simulink model "COSTEP"  (R2024b)
settings: Solver=FixedStepAuto  StartTime=0.0  StopTime=25  FixedStep=1/3600  RelTol=1e-3
model workspace (MAT data in the model file):
  AD : Simulink.Parameter (value not decoded)
  AG : Simulink.Parameter (value not decoded)
  AH : Simulink.Parameter (value not decoded)
  AV : Simulink.Parameter (value not decoded)
  AVP : Simulink.Parameter (value not decoded)
  BCHL : Simulink.Parameter (value not decoded)
  BCHV : Simulink.Parameter (value not decoded)
  BD : Simulink.Parameter (value not decoded)
  BDIST : Simulink.Parameter (value not decoded)
  BG : Simulink.Parameter (value not decoded)
  BH : Simulink.Parameter (value not decoded)
  BVP : Simulink.Parameter (value not decoded)
  CD : Simulink.Parameter (value not decoded)
  CDIST : Simulink.Parameter (value not decoded)
  CG : Simulink.Parameter (value not decoded)
  CH : Simulink.Parameter (value not decoded)
  CVP : Simulink.Parameter (value not decoded)
  DDIST : Simulink.Parameter (value not decoded)
  DIST_CONST : Simulink.Parameter (value not decoded)
  ISV : Simulink.Parameter (value not decoded)
  TLAST : Simulink.Parameter (value not decoded)
  TNEXT : Simulink.Parameter (value not decoded)
  XMW : Simulink.Parameter (value not decoded)
  XNS : Simulink.Parameter (value not decoded)
  XNS2 : Simulink.Parameter (value not decoded)
  XNS3 : Simulink.Parameter (value not decoded)
  XNSADD : Simulink.Parameter (value not decoded)
  XNSE : Simulink.Parameter (value not decoded)
symbols that are objects in the model workspace (value not decoded): AD, AG, AH, AV, AVP, BD, BG, BH, BVP, CD, CG, CH, CVP, XMW, XNS, XNS2, XNS3, XNSE
undefined symbols (not defined in the file or in its folder): magnitude, msgbox, SETPT, XMEAS, XMV
libraries: mylib x381, dspindex x31
(part 8 of 12)

== system COSTEP/Control Mode/Braatz/ 3/CONTROL 4 ==
  XMEAS(4) : Inport
  SETPT(4) : Inport  Port=2
  P Control Velocity form : mylib/Braatz Control/P Control Velocity form  Kc=GAIN4  Ts=SI4  X_0=XMV4_0  H=HIGH4
  XMV(4) : Outport  VectorParamsAs1DForOutWhenUnconnected=off
  wires:
  P Control Velocity form/1 -> XMV(4)/1
  XMEAS(4)/1 -> P Control Velocity form/2
  SETPT(4)/1 -> P Control Velocity form/1

== system COSTEP/Control Mode/Braatz/ 4/CONTROL 5 ==
  XMEAS(5) : Inport
  Constant4 : Constant  Value=SETPT5
  PI Control Measurement Velocity form : mylib/Braatz Control/PI Control Measurement Velocity form  Kc=GAIN5  Ti=TAUI5  Ts=SI5  X_0=XMV5_0  H=HIGH5
  XMV(5) : Outport  VectorParamsAs1DForOutWhenUnconnected=off
  wires:
  XMEAS(5)/1 -> PI Control Measurement Velocity form/2
  PI Control Measurement Velocity form/1 -> XMV(5)/1
  Constant4/1 -> PI Control Measurement Velocity form/1

== system COSTEP/Control Mode/Braatz/ 5/CONTROL 7 ==
  XMEAS(12) : Inport
  Constant4 : Constant  Value=SETPT7
  P Control Velocity form : mylib/Braatz Control/P Control Velocity form  Kc=GAIN7  Ts=SI7  X_0=XMV7_0  H=HIGH7
  XMV(7) : Outport  VectorParamsAs1DForOutWhenUnconnected=off
  wires:
  P Control Velocity form/1 -> XMV(7)/1
  Constant4/1 -> P Control Velocity form/1
  XMEAS(12)/1 -> P Control Velocity form/2

== system COSTEP/Control Mode/Braatz/ 6/CONTROL 8 ==
  XMEAS(15) : Inport
  Constant4 : Constant  Value=SETPT8
  P Control Velocity form : mylib/Braatz Control/P Control Velocity form  Kc=GAIN8  Ts=SI8  X_0=XMV8_0  H=HIGH8
  XMV(8) : Outport  VectorParamsAs1DForOutWhenUnconnected=off
  wires:
  P Control Velocity form/1 -> XMV(8)/1
  Constant4/1 -> P Control Velocity form/1
  XMEAS(15)/1 -> P Control Velocity form/2

== system COSTEP/Control Mode/Braatz/ 7/CONTROL 11 ==
  XMEAS(17) : Inport
  Constant4 : Constant  Value=SETPT11
  PI Control Measurement Velocity form : mylib/Braatz Control/PI Control Measurement Velocity form  Kc=GAIN11  Ti=TAUI11  Ts=SI11  X_0=XMV11_0  H=HIGH11
  XMV(11) : Outport  VectorParamsAs1DForOutWhenUnconnected=off
  wires:
  PI Control Measurement Velocity form/1 -> XMV(11)/1
  Constant4/1 -> PI Control Measurement Velocity form/1
  XMEAS(17)/1 -> PI Control Measurement Velocity form/2

== system COSTEP/Control Mode/Braatz/ 8/CONTROL 10 ==
  XMEAS(21) : Inport
  SETPT(10) : Inport  Port=2
  PI Control Measurement Velocity form : mylib/Braatz Control/PI Control Measurement Velocity form  Kc=GAIN10  Ti=TAUI10  Ts=SI10  X_0=XMV10_0  H=HIGH10
  XMV(10) : Outport  VectorParamsAs1DForOutWhenUnconnected=off
  wires:
  PI Control Measurement Velocity form/1 -> XMV(10)/1
  SETPT(10)/1 -> PI Control Measurement Velocity form/1
  XMEAS(21)/1 -> PI Control Measurement Velocity form/2

== system COSTEP/Control Mode/Braatz/ 8/CONTROL 18 ==
  XMEAS(9) : Inport
  Constant : Constant  Value=SETPT18
  PI Control Setpoint Velocity form : mylib/Braatz Control/PI Control Setpoint Velocity form  Kc=GAIN18  Ti=TAUI18  Ts=SI18  X_0=SETPT10  H=HIGH10  HS=HIGH18
  SETPT(10) : Outport  VectorParamsAs1DForOutWhenUnconnected=off
  wires:
  Constant/1 -> PI Control Setpoint Velocity form/1
  XMEAS(9)/1 -> PI Control Setpoint Velocity form/2
  PI Control Setpoint Velocity form/1 -> SETPT(10)/1

== system COSTEP/Control Mode/Braatz/ 9/CONTROL 16 ==
  XMEAS(18) : Inport
  SETPT(16) : Inport  Port=2
  PI Control Setpoint Velocity form : mylib/Braatz Control/PI Control Setpoint Velocity form  Kc=GAIN16  Ti=TAUI16  Ts=SI16  X_0=SETPT9  H=HIGH9  HS=HIGH16
  SETPT(9) : Outport  VectorParamsAs1DForOutWhenUnconnected=off
  wires:
  SETPT(16)/1 -> PI Control Setpoint Velocity form/1
  XMEAS(18)/1 -> PI Control Setpoint Velocity form/2
  PI Control Setpoint Velocity form/1 -> SETPT(9)/1

== system COSTEP/Control Mode/Braatz/ 9/CONTROL 20 ==
  XMEAS(38) : Inport
  Constant : Constant  Value=SETPT20
  PI Control Setpoint Velocity form : mylib/Braatz Control/PI Control Setpoint Velocity form  Kc=GAIN20  Ti=TAUI20  Ts=SI20  X_0=SETPT16  H=HIGH16  HS=HIGH20
  SETPT(16) : Outport  VectorParamsAs1DForOutWhenUnconnected=off
  wires:
  Constant/1 -> PI Control Setpoint Velocity form/1
  XMEAS(38)/1 -> PI Control Setpoint Velocity form/2
  PI Control Setpoint Velocity form/1 -> SETPT(16)/1

== system COSTEP/Control Mode/Braatz/ 9/CONTROL 9 ==
  XMEAS(19) : Inport
  SETPT(9) : Inport  Port=2
  P Control Velocity form : mylib/Braatz Control/P Control Velocity form  Kc=GAIN9  Ts=SI9  X_0=XMV9_0  H=HIGH9
  XMV(9) : Outport  VectorParamsAs1DForOutWhenUnconnected=off
  wires:
  SETPT(9)/1 -> P Control Velocity form/1
  P Control Velocity form/1 -> XMV(9)/1
  XMEAS(19)/1 -> P Control Velocity form/2

== system COSTEP/Mixing Zone/Stream 6/Subsystem/If Action Subsystem ==
  In1 : Inport
  Action Port : ActionPort  ActionPortLabel=if(u1 < 0)
  Out1 : Outport  VectorParamsAs1DForOutWhenUnconnected=off
  wires:
  In1/1 -> Out1/1

== system COSTEP/Mixing Zone/Stream 6/Subsystem/If Action Subsystem1 ==
  In1 : Inport
  Action Port : ActionPort  ActionPortLabel=else
  Out1 : Outport  VectorParamsAs1DForOutWhenUnconnected=off
  wires:
  In1/1 -> Out1/1

== system COSTEP/Process Measurements/Feed Streams/D Feed/XMWS(1) Molecular weight of Stream 1 lb//lb-mol ==
  XST(I,1) : Inport
  Product : Product
  Sum of Elements : Sum  Inputs=+
  "XMW(I) Molecular weight of components lb/lb-mol " : Constant  Value=XMW
  XMWS(1) : Outport  VectorParamsAs1DForOutWhenUnconnected=off
  wires:
  Sum of Elements/1 -> XMWS(1)/1
  Product/1 -> Sum of Elements/1
  XST(I,1)/1 -> Product/1
  "XMW(I) Molecular weight of components lb/lb-mol "/1 -> Product/2

== system COSTEP/Process Measurements/Feed Streams/E Feed/XMWS(2) Molecular weight of Stream 2 lb//lb-mol ==
  XST(I,2) : Inport
  Product : Product
  Sum of Elements : Sum  Inputs=+
  "XMW(I) Molecular weight of components lb/lb-mol " : Constant  Value=XMW
  XMWS(2) : Outport  VectorParamsAs1DForOutWhenUnconnected=off
  wires:
  Sum of Elements/1 -> XMWS(2)/1
  Product/1 -> Sum of Elements/1
  XST(I,2)/1 -> Product/1
  "XMW(I) Molecular weight of components lb/lb-mol "/1 -> Product/2

== system COSTEP/Process Measurements/Product analysis/Subsystem/Subsystem ==
  XST : Inport
  Constant : Constant  Value=100
  Multiport Selector : dspindex/Multiport Selector  rowsOrCols=Rows  idxCellArray={4,5,6,7,8}  idxErrMode=Clip Index
  XCMP(37) : Product
  XCMP(38) : Product
  XCMP(39) : Product
  XCMP(40) : Product
  XCMP(41) : Product
  "XCMP(37) " : Outport  VectorParamsAs1DForOutWhenUnconnected=off
  "XCMP(38) " : Outport  Port=2  VectorParamsAs1DForOutWhenUnconnected=off
  "XCMP(39) " : Outport  Port=3  VectorParamsAs1DForOutWhenUnconnected=off
  "XCMP(40) " : Outport  Port=4  VectorParamsAs1DForOutWhenUnconnected=off
  "XCMP(41) " : Outport  Port=5  VectorParamsAs1DForOutWhenUnconnected=off
  wires:
  Constant/1 -> XCMP(38)/2, XCMP(40)/2, XCMP(41)/2, XCMP(39)/2, XCMP(37)/2
  Multiport Selector/1 -> XCMP(37)/1
  XCMP(37)/1 -> "XCMP(37) "/1  "XCMP(37)"
  Multiport Selector/5 -> XCMP(41)/1
  XCMP(39)/1 -> "XCMP(39) "/1  "XCMP(39)"
  XST/1 -> Multiport Selector/1
  Multiport Selector/4 -> XCMP(40)/1
  Multiport Selector/2 -> XCMP(38)/1
  Multiport Selector/3 -> XCMP(39)/1
  XCMP(38)/1 -> "XCMP(38) "/1  "XCMP(38)"
  XCMP(41)/1 -> "XCMP(41) "/1  "XCMP(41)"
  XCMP(40)/1 -> "XCMP(40) "/1  "XCMP(40)"

== system COSTEP/Process Measurements/Purge gas analysis/Subsystem/Subsystem ==
  XST : Inport
  Constant : Constant  Value=100
  Multiport Selector : dspindex/Multiport Selector  rowsOrCols=Rows  idxCellArray={ 1,2,3,4,5,6,7,8}  idxErrMode=Clip Index
  XCMP(29) : Product
  XCMP(30) : Product
  XCMP(31) : Product
  XCMP(32) : Product
  XCMP(33) : Product
  XCMP(34) : Product
  XCMP(35) : Product
  XCMP(36) : Product
  "XCMP(29) " : Outport  VectorParamsAs1DForOutWhenUnconnected=off
  "XCMP(30) " : Outport  Port=2  VectorParamsAs1DForOutWhenUnconnected=off
  "XCMP(31) " : Outport  Port=3  VectorParamsAs1DForOutWhenUnconnected=off
  "XCMP(32) " : Outport  Port=4  VectorParamsAs1DForOutWhenUnconnected=off
  "XCMP(33) " : Outport  Port=5  VectorParamsAs1DForOutWhenUnconnected=off
  "XCMP(34) " : Outport  Port=6  VectorParamsAs1DForOutWhenUnconnected=off
  "XCMP(35) " : Outport  Port=7  VectorParamsAs1DForOutWhenUnconnected=off
  "XCMP(36) " : Outport  Port=8  VectorParamsAs1DForOutWhenUnconnected=off
  wires:
  XCMP(32)/1 -> "XCMP(32) "/1  "XCMP(32)"
  Multiport Selector/6 -> XCMP(34)/1
  Multiport Selector/8 -> XCMP(36)/1
  XCMP(29)/1 -> "XCMP(29) "/1  "XCMP(29)"
  Multiport Selector/5 -> XCMP(33)/1
  Multiport Selector/7 -> XCMP(35)/1
  XCMP(30)/1 -> "XCMP(30) "/1  "XCMP(30)"
  Multiport Selector/1 -> XCMP(29)/1
  Multiport Selector/3 -> XCMP(31)/1
  Constant/1 -> XCMP(32)/2, XCMP(36)/2, XCMP(35)/2, XCMP(34)/2, XCMP(33)/2, XCMP(31)/2, XCMP(30)/2, XCMP(29)/2
  XCMP(33)/1 -> "XCMP(33) "/1  "XCMP(33)"
  Multiport Selector/4 -> XCMP(32)/1
  XST/1 -> Multiport Selector/1
  Multiport Selector/2 -> XCMP(30)/1
  XCMP(31)/1 -> "XCMP(31) "/1  "XCMP(31)"
  XCMP(35)/1 -> "XCMP(35) "/1  "XCMP(35)"
  XCMP(36)/1 -> "XCMP(36) "/1  "XCMP(36)"
  XCMP(34)/1 -> "XCMP(34) "/1  "XCMP(34)"

== system COSTEP/Process Measurements/Reactor feed analysis/Subsystem/Subsystem ==
  XST : Inport
  Constant : Constant  Value=100
  Multiport Selector : dspindex/Multiport Selector  rowsOrCols=Rows  idxCellArray={ 1,2,3,4,5,6,}  idxErrMode=Clip Index
  XCMP(23) : Product
  XCMP(24) : Product
  XCMP(25) : Product
  XCMP(26) : Product
  XCMP(27) : Product
  XCMP(28) : Product
  XCMP(23)1 : Outport  VectorParamsAs1DForOutWhenUnconnected=off
  XCMP(24)1 : Outport  Port=2  VectorParamsAs1DForOutWhenUnconnected=off
  XCMP(25)1 : Outport  Port=3  VectorParamsAs1DForOutWhenUnconnected=off
  XCMP(26)1 : Outport  Port=4  VectorParamsAs1DForOutWhenUnconnected=off
  XCMP(27)1 : Outport  Port=5  VectorParamsAs1DForOutWhenUnconnected=off
  XCMP(28)1 : Outport  Port=6  VectorParamsAs1DForOutWhenUnconnected=off
  wires:
  Multiport Selector/1 -> XCMP(23)/1  "XST(1;7)"
  Multiport Selector/4 -> XCMP(26)/1  "XST(4;7)"
  Constant/1 -> XCMP(26)/2, XCMP(28)/2, XCMP(27)/2, XCMP(25)/2, XCMP(24)/2, XCMP(23)/2
  Multiport Selector/2 -> XCMP(24)/1  "XST(2;7)"
  XST/1 -> Multiport Selector/1
  Multiport Selector/6 -> XCMP(28)/1  "XST(6:7)"
  Multiport Selector/3 -> XCMP(25)/1  "XST(3;7)"
  XCMP(23)/1 -> XCMP(23)1/1  "XCMP(23)"
  Multiport Selector/5 -> XCMP(27)/1  "XST(5;7)"
  XCMP(25)/1 -> XCMP(25)1/1  "XCMP(25)"
  XCMP(26)/1 -> XCMP(26)1/1  "XCMP(26)"
  XCMP(24)/1 -> XCMP(24)1/1  "XCMP(24)"
  XCMP(27)/1 -> XCMP(27)1/1  "XCMP(27)"
  XCMP(28)/1 -> XCMP(28)1/1  "XCMP(28)"

== system COSTEP/Random number generator/Stream Measurements SMEAS Gas analysis1/Gas Analysis Delay/Subsystem ==
  In1 : Inport
  In2 : Inport  Port=2
  If : If  NumInputs=2  IfExpression=u1 == u2
  If Action Subsystem : Subsystem  TreatAsAtomicUnit=on
  If Action Subsystem1 : Subsystem  TreatAsAtomicUnit=on
  Rounding Function : Rounding  Operator=round
  Out1 : Outport  VectorParamsAs1DForOutWhenUnconnected=off
  Out2 : Outport  Port=2  VectorParamsAs1DForOutWhenUnconnected=off
  wires:
  Rounding Function/1 -> If/1, If Action Subsystem1/1(In1)
  In2/1 -> If/2
  If Action Subsystem/1(Out1) -> Out1/1
  If Action Subsystem1/1(Out1) -> Out2/1
  In1/1 -> Rounding Function/1
  If/1 -> If Action Subsystem/Action
  If/2 -> If Action Subsystem1/Action

== system COSTEP/Random number generator/Stream Measurements SMEAS Gas analysis1/If Action Subsystem3/Subsystem ==
  G : Inport
  Bus Creator2 : BusCreator  Inputs=9
  Stream 1 : Subsystem
  Stream 13 : Subsystem
  Stream 2 : Subsystem
  Stream 3 : Subsystem
  Stream 4 : Subsystem
  Stream 5 : Subsystem
  Stream 6 : Subsystem
  Stream 8 : Subsystem
  Stream 9 : Subsystem
  XMNSE2 : Outport  VectorParamsAs1DForOutWhenUnconnected=off
  G_NEW : Outport  Port=2  VectorParamsAs1DForOutWhenUnconnected=off
  wires:
  Bus Creator2/1 -> XMNSE2/1
  G/1 -> Stream 1/1(G)
  Stream 1/1(Stream 1) -> Bus Creator2/1
  Stream 1/2(G_NEW) -> Stream 2/1(G)
  Stream 2/1(Stream 2) -> Bus Creator2/2
  Stream 2/2(G_NEW) -> Stream 3/1(G)
  Stream 3/1(Stream 3) -> Bus Creator2/3
  Stream 3/2(G_NEW) -> Stream 4/1(G)
  Stream 4/1(Stream 4) -> Bus Creator2/4
  Stream 4/2(G_NEW) -> Stream 5/1(G)
  Stream 5/1(Stream 5) -> Bus Creator2/5
  Stream 5/2(G_NEW) -> Stream 6/1(G)
  Stream 6/1(Stream 6) -> Bus Creator2/6
  Stream 6/2(G_NEW) -> Stream 8/1(G)
  Stream 8/1(Stream 8) -> Bus Creator2/7
  Stream 8/2(G_NEW) -> Stream 9/1(G)
  Stream 9/1(Stream 9) -> Bus Creator2/8
  Stream 9/2(G_NEW) -> Stream 13/1(G)
  Stream 13/2(G_NEW) -> G_NEW/1
  Stream 13/1(Stream 13) -> Bus Creator2/9

== system COSTEP/Random number generator/Stream Measurements SMEAS Gas analysis1/Subsystem/If Action Subsystem ==
  In1 : Inport
  Action Port : ActionPort  ActionPortLabel=if(u1 == 0)
  Out1 : Outport  VectorParamsAs1DForOutWhenUnconnected=off
  wires:
  In1/1 -> Out1/1

== system COSTEP/Random number generator/Stream Measurements SMEAS Gas analysis1/Subsystem/If Action Subsystem1 ==
  In1 : Inport
  Action Port : ActionPort  ActionPortLabel=else
  Out1 : Outport  VectorParamsAs1DForOutWhenUnconnected=off
  wires:
  In1/1 -> Out1/1

== system COSTEP/Random number generator/Stream Measurements SMEAS Product analysis1/Gas Analysis Delay/Subsystem ==
  In1 : Inport
  In2 : Inport  Port=2
  If : If  NumInputs=2  IfExpression=u1 == u2
  If Action Subsystem : Subsystem  TreatAsAtomicUnit=on
  If Action Subsystem1 : Subsystem  TreatAsAtomicUnit=on
  Rounding Function : Rounding  Operator=round
  Out1 : Outport  VectorParamsAs1DForOutWhenUnconnected=off
  Out2 : Outport  Port=2  VectorParamsAs1DForOutWhenUnconnected=off
  wires:
  Rounding Function/1 -> If/1, If Action Subsystem1/1(In1)
  In2/1 -> If/2
  If Action Subsystem/1(Out1) -> Out1/1
  If Action Subsystem1/1(Out1) -> Out2/1
  In1/1 -> Rounding Function/1
  If/1 -> If Action Subsystem/Action
  If/2 -> If Action Subsystem1/Action

== system COSTEP/Random number generator/Stream Measurements SMEAS Product analysis1/If Action Subsystem3/Subsystem ==
  G : Inport
  Bus Creator : BusCreator  Inputs=2
  Subsystem1 : Subsystem
  Subsystem2 : Subsystem
  XMNSE3 : Outport  VectorParamsAs1DForOutWhenUnconnected=off
  G_NEW : Outport  Port=2  VectorParamsAs1DForOutWhenUnconnected=off
  wires:
  G/1 -> Subsystem1/1(G)
  Subsystem1/1(Stream 11) -> Bus Creator/1
  Bus Creator/1 -> XMNSE3/1
  Subsystem1/2(G_NEW) -> Subsystem2/1(G)
  Subsystem2/1(Stream 13) -> Bus Creator/2
  Subsystem2/2(G_NEW) -> G_NEW/1

== system COSTEP/Random number generator/Stream Measurements SMEAS Product analysis1/Subsystem/If Action Subsystem ==
  In1 : Inport
  Action Port : ActionPort  ActionPortLabel=if(u1 == 0)
  Out1 : Outport  VectorParamsAs1DForOutWhenUnconnected=off
  wires:
  In1/1 -> Out1/1

== system COSTEP/Random number generator/Stream Measurements SMEAS Product analysis1/Subsystem/If Action Subsystem1 ==
  In1 : Inport
  Action Port : ActionPort  ActionPortLabel=else
  Out1 : Outport  VectorParamsAs1DForOutWhenUnconnected=off
  wires:
  In1/1 -> Out1/1

== system COSTEP/Reactor/Reaction Rates/Component reaction rate lb-mol//h/Subsystem ==
  RR : Inport
  " " : Sum  Inputs=---
  Bus Selector : BusSelector  OutputSignals=RR(1),RR(2),RR(3)
  CRXR(1) : Outport  VectorParamsAs1DForOutWhenUnconnected=off
  wires:
  " "/1 -> CRXR(1)/1  "CRXR(1)"
  Bus Selector/2 -> " "/2  "<RR(2)>"
  Bus Selector/3 -> " "/3  "<RR(3)>"
  RR/1 -> Bus Selector/1
  Bus Selector/1 -> " "/1  "<RR(1)>"

== system COSTEP/Reactor/Reaction Rates/Component reaction rate lb-mol//h/Subsystem1 ==
  RR : Inport
  " " : Sum  Inputs=--
  Bus Selector : BusSelector  OutputSignals=RR(1),RR(2)
  CRXR(3) : Outport  VectorParamsAs1DForOutWhenUnconnected=off
  wires:
  " "/1 -> CRXR(3)/1  "CRXR(3)"
  RR/1 -> Bus Selector/1
  Bus Selector/1 -> " "/1  "<RR(1)>"
  Bus Selector/2 -> " "/2  "<RR(2)>"

== system COSTEP/Reactor/Reaction Rates/Component reaction rate lb-mol//h/Subsystem2 ==
  RR : Inport
  " " : Sum  Inputs=--
  Bus Selector : BusSelector  OutputSignals=RR(1),RR(4)
  Gain : Gain  Gain=1.5
  CRXR(4) : Outport  VectorParamsAs1DForOutWhenUnconnected=off
  wires:
  Gain/1 -> " "/2
  Bus Selector/1 -> " "/1  "<RR(1)>"
  " "/1 -> CRXR(4)/1  "CRXR(4)"
  RR/1 -> Bus Selector/1
  Bus Selector/2 -> Gain/1  "<RR(4)>"

== system COSTEP/Reactor/Reaction Rates/Component reaction rate lb-mol//h/Subsystem3 ==
  RR : Inport
  " " : Sum  Inputs=--
  Bus Selector : BusSelector  OutputSignals=RR(2),RR(3)
  CRXR(5) : Outport  VectorParamsAs1DForOutWhenUnconnected=off
  wires:
  " "/1 -> CRXR(5)/1  "CRXR(5)"
  RR/1 -> Bus Selector/1
  Bus Selector/1 -> " "/1  "<RR(2)>"
  Bus Selector/2 -> " "/2  "<RR(3)>"

== system COSTEP/Reactor/Reaction Rates/Component reaction rate lb-mol//h/Subsystem4 ==
  RR : Inport
  " " : Sum
  Bus Selector : BusSelector  OutputSignals=RR(3),RR(4)
  CRXR(6) : Outport  VectorParamsAs1DForOutWhenUnconnected=off
  wires:
  " "/1 -> CRXR(6)/1  "CRXR(6)"
  RR/1 -> Bus Selector/1
  Bus Selector/2 -> " "/2  "<RR(4)>"
  Bus Selector/1 -> " "/1  "<RR(3)>"

== system COSTEP/Reactor/Reaction Rates/Component reaction rate lb-mol//h/Subsystem5 ==
  RR : Inport
  Bus Selector : BusSelector  OutputSignals=RR(1)
  Gain : Gain
  CRXR(7) : Outport  VectorParamsAs1DForOutWhenUnconnected=off
  wires:
  Bus Selector/1 -> Gain/1  "<RR(1)>"
  RR/1 -> Bus Selector/1
  Gain/1 -> CRXR(7)/1  "CRXR(7)"

== system COSTEP/Reactor/Reaction Rates/Component reaction rate lb-mol//h/Subsystem6 ==
  RR : Inport
  " " : Gain
  Bus Selector : BusSelector  OutputSignals=RR(2)
  CRXR(8) : Outport  VectorParamsAs1DForOutWhenUnconnected=off
  wires:
  " "/1 -> CRXR(8)/1  "CRXR(8)"
  RR/1 -> Bus Selector/1
  Bus Selector/1 -> " "/1  "<RR(2)>"

== system COSTEP/Reactor/Reaction Rates/Reaction rates lb-mol//h/ Reaction rate of reaction 4 lb-mol//ft3·h     ==
  PPR : Inport
  TKR : Inport  Port=2
  Activation energy cal/mol : Constant  Value=60000
  Bus Selector : BusSelector  OutputSignals=PPR(1),PPR(4)
  Divide : Product  Inputs=*//
  Divide1 : Product  Inputs=3
  Gain : Gain  Gain=0.767488334
  Math Function2 : Math  SignedPower=on
  Preexponential factor lb-mol/ft3·h·mmHg : Constant  Value=53.4060443
  Subtract : Sum  Inputs=+-
  Universal gas constant cal/mol·K : Constant  Value=1.987
  RR(4) : Outport  VectorParamsAs1DForOutWhenUnconnected=off
  wires:
  Divide/1 -> Subtract/2
  Universal gas constant cal/mol·K/1 -> Divide/2
  Preexponential factor lb-mol/ft3·h·mmHg/1 -> Subtract/1
  Activation energy cal/mol/1 -> Divide/1
  TKR/1 -> Divide/3
  Subtract/1 -> Math Function2/1
  Divide1/1 -> RR(4)/1
  Bus Selector/2 -> Divide1/3  "<PPR(4)>"
  Gain/1 -> Divide1/1
  Math Function2/1 -> Gain/1
  PPR/1 -> Bus Selector/1
  Bus Selector/1 -> Divide1/2  "<PPR(1)>"

== system COSTEP/Reactor/Reaction Rates/Reaction rates lb-mol//h/Reaction rate of reaction 1 lb-mol//ft3·h ==
  PPR : Inport
  TKR : Inport  Port=2
  " " : Constant  Value=0
  Abs : Abs  SaturateOnIntegerOverflow=off
  Bus Selector : BusSelector  OutputSignals=PPR(1),PPR(3)
  If : If  NumInputs=2  IfExpression=u1>0 & u2>0
  If Action Subsystem : Subsystem  TreatAsAtomicUnit=on
  If Action Subsystem2 : Subsystem  TreatAsAtomicUnit=on
  Merge1 : Merge
  "RR(1) Reaction rate of 1st reaction lb-mol/ft3·h " : Subsystem
  RR(1) : Outport  VectorParamsAs1DForOutWhenUnconnected=off
  wires:
  "RR(1) Reaction rate of 1st reaction lb-mol/ft3·h "/1(RR(1)) -> If Action Subsystem/1(In1)
  If/1 -> If Action Subsystem/Action
  " "/1 -> If Action Subsystem2/1(In1)
  If/2 -> If Action Subsystem2/Action
  Merge1/1 -> Abs/1
  If Action Subsystem/1(Out1) -> Merge1/1
  If Action Subsystem2/1(Out1) -> Merge1/2
  TKR/1 -> "RR(1) Reaction rate of 1st reaction lb-mol/ft3·h "/2(TKR)
  Abs/1 -> RR(1)/1
  PPR/1 -> "RR(1) Reaction rate of 1st reaction lb-mol/ft3·h "/1(PPR), Bus Selector/1
  Bus Selector/1 -> If/1  "<PPR(1)>"
  Bus Selector/2 -> If/2  "<PPR(3)>"

== system COSTEP/Reactor/Reaction Rates/Reaction rates lb-mol//h/Reaction rate of reaction 2 lb-mol//ft3·h ==
  PPR : Inport
  TKR : Inport  Port=2
  " " : Constant  Value=0
  Abs : Abs  SaturateOnIntegerOverflow=off
  Bus Selector : BusSelector  OutputSignals=PPR(1),PPR(3)
  If : If  NumInputs=2  IfExpression=u1>0 & u2>0
  If Action Subsystem : Subsystem  TreatAsAtomicUnit=on
  If Action Subsystem2 : Subsystem  TreatAsAtomicUnit=on
  Merge1 : Merge
  "RR(2) Reaction rate of 2nd reaction lb-mol/ft3·h " : Subsystem
  RR(2) : Outport  VectorParamsAs1DForOutWhenUnconnected=off
  wires:
  If/1 -> If Action Subsystem/Action
  If/2 -> If Action Subsystem2/Action
  "RR(2) Reaction rate of 2nd reaction lb-mol/ft3·h "/1(RR(2)) -> If Action Subsystem/1(In1)
  " "/1 -> If Action Subsystem2/1(In1)
  If Action Subsystem2/1(Out1) -> Merge1/2
  TKR/1 -> "RR(2) Reaction rate of 2nd reaction lb-mol/ft3·h "/2(TKR)
  If Action Subsystem/1(Out1) -> Merge1/1
  Merge1/1 -> Abs/1
  Abs/1 -> RR(2)/1
  PPR/1 -> "RR(2) Reaction rate of 2nd reaction lb-mol/ft3·h "/1(PPR), Bus Selector/1
  Bus Selector/1 -> If/1  "<PPR(1)>"
  Bus Selector/2 -> If/2  "<PPR(3)>"

== system COSTEP/Reactor/Reaction Rates/Reaction rates lb-mol//h/Reaction rate of reaction 3 lb-mol//ft3·h   ==
  PPR : Inport
  TKR : Inport  Port=2
  Activation energy cal/mol : Constant  Value=60000
  Bus Selector : BusSelector  OutputSignals=PPR(1),PPR(5)
  Divide : Product  Inputs=*//
  Divide1 : Product  Inputs=3
  Math Function2 : Math  SignedPower=on
  Preexponential factor lb-mol/ft3·h·mmHg : Constant  Value=53.4060443
  Subtract : Sum  Inputs=+-
  Universal gas constant cal/mol·K : Constant  Value=1.987
  RR(3) : Outport  VectorParamsAs1DForOutWhenUnconnected=off
  wires:
  Divide/1 -> Subtract/2
  Universal gas constant cal/mol·K/1 -> Divide/2
  Preexponential factor lb-mol/ft3·h·mmHg/1 -> Subtract/1
  Activation energy cal/mol/1 -> Divide/1
  TKR/1 -> Divide/3
  Subtract/1 -> Math Function2/1
  Bus Selector/2 -> Divide1/3  "<PPR(5)>"
  Divide1/1 -> RR(3)/1
  Math Function2/1 -> Divide1/1
  PPR/1 -> Bus Selector/1
  Bus Selector/1 -> Divide1/2  "<PPR(1)>"

== system COSTEP/Reactor/Reactor Heat exchanger/Position of Valve 12 %/Control valve ==
  XMV(12) : Inport
  Saturation : Saturate  UpperLimit=100  LowerLimit=0
  VCV(12) : Outport  PortDimensions=1  VectorParamsAs1DForOutWhenUnconnected=off
  wires:
  Saturation/1 -> VCV(12)/1
  XMV(12)/1 -> Saturation/1

== system COSTEP/Reactor/Reactor Heat exchanger/Reactor Heat exchanger/AGSP Agitation speed ==
  VPOS(12) : Inport
  " " : Product  Inputs=*/
  Add : Sum
  Constant1 : Constant  Value=150
  Constant2 : Constant  Value=100
  AGSP : Outport  VectorParamsAs1DForOutWhenUnconnected=off
  wires:
  Constant2/1 -> " "/2
  " "/1 -> AGSP/1
  VPOS(12)/1 -> Add/1
  Constant1/1 -> Add/2
  Add/1 -> " "/1

== system COSTEP/Reactor/Reactor Heat exchanger/Reactor Heat exchanger/Cooling water outlet temperature ==
  FWR : Inport
  QUR : Inport  Port=2  PortDimensions=1
  Constant : Constant  Value=37
  Constant1 : Constant  Value=1e6
  Constant2 : Constant  Value=1.8
  Constant6 : Constant  Value=500.53
  Divide : Product  Inputs=*/
  Divide1 : Product
  Divide2 : Product  Inputs=*/
  HWR : Constant  Value=7060
  Initial state variable : mylib/Initial state variable
  Integration : mylib/Integration  SystemSampleTime=-1  VariantActivationTime=update diagram  AllowFlexibleInterface=on  Latency=0  AutoFrameSizeCalculation=off
  Product : Product  Inputs=3
  Subtract : Sum  Inputs=+-
  "TCWR Inlet temperature of cooling water °C " : Subsystem
  TCWR-TWR : Sum  Inputs=+-
  "YY(37) " : Outport  VectorParamsAs1DForOutWhenUnconnected=off
  tag scope: TCWR=global, TWR=global
  wires:
  Divide2/1 -> Integration/1
  Initial state variable/1 -> Integration/2
  "TCWR Inlet temperature of cooling water °C "/1(TCWR) -> [TCWR], TCWR-TWR/1
  Integration/1 -> TCWR-TWR/2, "YY(37) "/1, [TWR]
  FWR/1 -> Product/1
  Constant6/1 -> Product/2
  TCWR-TWR/1 -> Product/3
  QUR/1 -> Divide1/1
  Constant1/1 -> Divide1/2
  Divide1/1 -> Divide/1
  Constant2/1 -> Divide/2
  Product/1 -> Subtract/1
  Divide/1 -> Subtract/2
  Subtract/1 -> Divide2/1
  HWR/1 -> Divide2/2
  Constant/1 -> Initial state variable/1

== system COSTEP/Reactor/Reactor Heat exchanger/Reactor Heat exchanger/FWR Flow of cooling water to reactor gallons per minute ==
  VPOS(10) : Inport
  VRNG(10) : Inport  Port=2
  " " : Product  Inputs=**/
  Constant2 : Constant  Value=100
  FWR : Outport  VectorParamsAs1DForOutWhenUnconnected=off
  wires:
  Constant2/1 -> " "/3
  " "/1 -> FWR/1
  VPOS(10)/1 -> " "/1
  VRNG(10)/1 -> " "/2

== system COSTEP/Reactor/Reactor Heat exchanger/Reactor Heat exchanger/Subsystem ==
  VLR : Inport
  Constant : Constant  Value=7.8
  Constant1 : Constant
  Constant2 : Constant  Value=0
  Constant3 : Constant  Value=0.025
  Constant4 : Constant  Value=0.25
  Divide : Product  Inputs=*/
  Divide1 : Product  Inputs=**
  If : If  IfExpression=u1 > 50  ElseIfExpressions=u1 < 10
  If Action Subsystem : Subsystem  TreatAsAtomicUnit=on
  If Action Subsystem1 : Subsystem  TreatAsAtomicUnit=on
  If Action Subsystem2 : Subsystem  TreatAsAtomicUnit=on
  Subtract : Sum  Inputs=+-
  UARLEV : Merge  Inputs=3
  "UARLEV " : Outport  VectorParamsAs1DForOutWhenUnconnected=off
  wires:
  If/2 -> If Action Subsystem1/Action
  If/1 -> If Action Subsystem/Action
  UARLEV/1 -> "UARLEV "/1
  If Action Subsystem1/1(Out1) -> UARLEV/2
  If Action Subsystem/1(Out1) -> UARLEV/1
  If/3 -> If Action Subsystem2/Action
  If Action Subsystem2/1(Out1) -> UARLEV/3
  VLR/1 -> Divide/1
  Constant/1 -> Divide/2
  Divide/1 -> Divide1/2, If/1
  Constant1/1 -> If Action Subsystem/1(In1)
  Constant2/1 -> If Action Subsystem1/1(In1)
  Constant3/1 -> Divide1/1
  Divide1/1 -> Subtract/1
  Constant4/1 -> Subtract/2
  Subtract/1 -> If Action Subsystem2/1(In1)

== system COSTEP/Reactor/Reactor Heat exchanger/Reactor Heat exchanger/Subsystem2 ==
  UARLEV : Inport
  AGSP : Inport  Port=2
  Add : Sum  Inputs=++-
  Constant : Constant  Value=-0.5
  Constant1 : Constant  Value=2.75
  Constant2 : Constant  Value=2.5
  Constant3 : Constant  Value=855490E-6
  Math Function : Math  Operator=magnitude^2  SignedPower=on
  Product : Product
  Product1 : Product
  UAR : Product  Inputs=3
  "UAR " : Outport
  wires:
  Constant/1 -> Product/1
  Constant3/1 -> UAR/3
  AGSP/1 -> Product1/2, Math Function/1
  Add/1 -> UAR/2
  Product1/1 -> Add/2
  Math Function/1 -> Product/2
  Constant1/1 -> Product1/1
  Constant2/1 -> Add/3
  Product/1 -> Add/1
  UAR/1 -> "UAR "/1
  UARLEV/1 -> UAR/1

== system COSTEP/Reactor/Reactor Heat exchanger/Reactor Heat exchanger/Subsystem3 ==
  UAR : Inport
  TWR : Inport  Port=2
  TCR : Inport  Port=3
  Bus Selector : BusSelector  OutputSignals=signal2.TESUB8(10)
  Constant4 : Constant
  Constant5 : Constant  Value=0.35
  Product2 : Product
  QUR : Product  Inputs=3
  Subtract : Sum  Inputs=+-
  Subtract1 : Sum  Inputs=+-
  "QUR " : Outport
  wires:
  Product2/1 -> Subtract1/2
  UAR/1 -> QUR/1
  Subtract/1 -> QUR/2
  [TESUB8] -> Bus Selector/1
  Constant4/1 -> Subtract1/1
  Subtract1/1 -> QUR/3
  Constant5/1 -> Product2/1
  TWR/1 -> Subtract/1
  Bus Selector/1 -> Product2/2  "<TESUB8(10)>"
  TCR/1 -> Subtract/2
  QUR/1 -> "QUR "/1

== system COSTEP/Reactor/Stream 8/Subsystem/If Action Subsystem ==
  In1 : Inport
  Action Port : ActionPort  ActionPortLabel=if(u1 < 0)
  Out1 : Outport  VectorParamsAs1DForOutWhenUnconnected=off
  wires:
  In1/1 -> Out1/1

== system COSTEP/Reactor/Stream 8/Subsystem/If Action Subsystem1 ==
  In1 : Inport
  Action Port : ActionPort  ActionPortLabel=else
  Out1 : Outport  VectorParamsAs1DForOutWhenUnconnected=off
  wires:
  In1/1 -> Out1/1

== system COSTEP/Reactor/Volume of Reactor/DLR Molar Density of Liquids in Reactor lb-mol//ft³    /DLR Molar Density of Liquids in Reactor lb-mol//ft³  ==
  X : Inport
  T : Inport  Port=2
  "  " : Constant
  "    " : Product  Inputs=*/
  AD(I) : Constant  Value=AD
  Add2 : Sum
  BD(I) : Constant  Value=BD
  CD(I) : Constant  Value=CD
  Liquid Density of Components lb/ft³ : Sum
  Molecular weight of components lb/lb-mol : Constant  Value=XMW
  Product : Product
  Product1 : Product
  Product2 : Product
  Sum of Elements : Sum  Inputs=+
  V Molar Volume of Components ft³/lb-mol : Product  Inputs=*/
  "R " : Outport  VectorParamsAs1DForOutWhenUnconnected=off
  wires:
  Liquid Density of Components lb/ft³/1 -> V Molar Volume of Components ft³/lb-mol/2
  Product1/1 -> Liquid Density of Components lb/ft³/2
  T/1 -> Product1/2, Product/2
  "  "/1 -> "    "/1
  AD(I)/1 -> Liquid Density of Components lb/ft³/1
  Add2/1 -> Product1/1
  V Molar Volume of Components ft³/lb-mol/1 -> Sum of Elements/1
  CD(I)/1 -> Product/1
  Product2/1 -> V Molar Volume of Components ft³/lb-mol/1
  BD(I)/1 -> Add2/1
  Product/1 -> Add2/2
  "    "/1 -> "R "/1
  X/1 -> Product2/1
  Sum of Elements/1 -> "    "/2
  Molecular weight of components lb/lb-mol/1 -> Product2/2

== system COSTEP/Separator/Stream 10/Subsystem/If Action Subsystem ==
  In1 : Inport
  Action Port : ActionPort  ActionPortLabel=if(u1 < 0)
  Out1 : Outport  VectorParamsAs1DForOutWhenUnconnected=off
  wires:
  In1/1 -> Out1/1

== system COSTEP/Separator/Stream 10/Subsystem/If Action Subsystem1 ==
  In1 : Inport
  Action Port : ActionPort  ActionPortLabel=else
  Out1 : Outport  VectorParamsAs1DForOutWhenUnconnected=off
  wires:
  In1/1 -> Out1/1

== system COSTEP/Separator/Stream 11/PTSL Pressure of Liquid From Separator mmHg/VPR Vapour Pressure mmHg ==
  TCR : Inport
  AVP(I) Antoine Coefficient A ln(mmHg) : Constant  Value=AVP
  Add : Sum
  Add1 : Sum
  BVP(I) Antoine Coefficient B ln(mmHg)·°C : Constant  Value=BVP
  CVP(I) Antoine Coefficient C °C : Constant  Value=CVP
  Divide : Product  Inputs=*/
  Math Function : Math  SignedPower=on
  VPR : Outport  VectorParamsAs1DForOutWhenUnconnected=off
  wires:
  BVP(I) Antoine Coefficient B ln(mmHg)·°C/1 -> Divide/1
  CVP(I) Antoine Coefficient C °C/1 -> Add/1
  AVP(I) Antoine Coefficient A ln(mmHg)/1 -> Add1/1
  Add/1 -> Divide/2
  Divide/1 -> Add1/2
  Add1/1 -> Math Function/1
  Math Function/1 -> VPR/1
  TCR/1 -> Add/2

== system COSTEP/Separator/Stream 9/Subsystem/If Action Subsystem2 ==
  In1 : Inport
  Action Port : ActionPort  ActionPortLabel=if(u1 < 1E-3)
  Out1 : Outport  VectorParamsAs1DForOutWhenUnconnected=off
  wires:
  In1/1 -> Out1/1

== system COSTEP/Separator/Stream 9/Subsystem/If Action Subsystem3 ==
  In1 : Inport
  Action Port : ActionPort  ActionPortLabel=else
  Out1 : Outport  PortDimensions=1  VectorParamsAs1DForOutWhenUnconnected=off
  wires:
  In1/1 -> Out1/1

== system COSTEP/Separator/Stream 9/Subsystem/Pressure drop ==
  Constant : Constant  Value=0.0
  DLP : Sum  Inputs=+-
  DLP Pressure drop between separator and reactor : Merge
  If : If  IfExpression=u1 < 0
  If Action Subsystem : Subsystem  TreatAsAtomicUnit=on
  If Action Subsystem1 : Subsystem  TreatAsAtomicUnit=on
  "DLP " : Outport  VectorParamsAs1DForOutWhenUnconnected=off
  wires:
  DLP Pressure drop between separator and reactor/1 -> "DLP "/1
  [PTV] -> DLP/1
  Constant/1 -> If Action Subsystem/1(In1)
  DLP/1 -> If Action Subsystem1/1(In1), If/1
  If/2 -> If Action Subsystem1/Action
  If/1 -> If Action Subsystem/Action
  [PTS] -> DLP/2
  If Action Subsystem1/1(Out1) -> DLP Pressure drop between separator and reactor/2
  If Action Subsystem/1(Out1) -> DLP Pressure drop between separator and reactor/1

== system COSTEP/Separator/Volume of Separator/DLS Molar Density of Liquids in Reactor lb-mol//ft³    /DLS Molar Density of Liquids in Separator lb-mol//ft³  ==
  X : Inport
  T : Inport  Port=2
  "  " : Constant
  "    " : Product  Inputs=*/
  AD(I) : Constant  Value=AD
  Add2 : Sum
  BD(I) : Constant  Value=BD
  CD(I) : Constant  Value=CD
  Liquid Density of Components lb/ft³ : Sum
  Product : Product
  Product1 : Product
  Product2 : Product
  Sum of Elements : Sum  Inputs=+
  V Molar Volume of Components ft³/lb-mol : Product  Inputs=*/
  XMW : Constant  Value=XMW
  "R " : Outport  VectorParamsAs1DForOutWhenUnconnected=off
  wires:
  Liquid Density of Components lb/ft³/1 -> V Molar Volume of Components ft³/lb-mol/2
  Product1/1 -> Liquid Density of Components lb/ft³/2
  T/1 -> Product1/2, Product/2
  "  "/1 -> "    "/1
  AD(I)/1 -> Liquid Density of Components lb/ft³/1
  Add2/1 -> Product1/1
  V Molar Volume of Components ft³/lb-mol/1 -> Sum of Elements/1
  CD(I)/1 -> Product/1
  Product2/1 -> V Molar Volume of Components ft³/lb-mol/1
  BD(I)/1 -> Add2/1
  Product/1 -> Add2/2
  "    "/1 -> "R "/1
  X/1 -> Product2/1
  Sum of Elements/1 -> "    "/2
  XMW/1 -> Product2/2

== system COSTEP/Stream Measurements/Subsystem6/A and C feed stream/Composition measurement mol% ==
  XST : Inport
  XMNSE : Inport  Port=2
  Bus Creator : BusCreator  Inputs=3
  Subsystem : Subsystem
  SMEASX(4) : Outport
  wires:
  Subsystem/3(SMEASXC(4)) -> Bus Creator/3  "SMEASXC(4)"
  XST/1 -> Subsystem/1(XST)
  Subsystem/2(SMEASXB(4)) -> Bus Creator/2  "SMEASXB(4)"
  Subsystem/1(SMEASXA(4)) -> Bus Creator/1  "SMEASXA(4)"
  Bus Creator/1 -> SMEASX(4)/1  "SMEASX(4)"
  XMNSE/1 -> Subsystem/2(XMNSE)

== system COSTEP/Stream Measurements/Subsystem6/A and C feed stream/Flow measurement in kg//h ==
  XMEAS in kscmh : Inport
  XST : Inport  Port=2
  " " : Constant  Value=35.3145
  "  " : Constant  Value=0.359
  Convert from lb/h to kg/h : Constant  Value=0.454
  Product : Product  Inputs=3
  XMWS Molecular weight of Stream lb/lb-mol : Subsystem
  lb-mol/h : Product  Inputs=**/
  "SMEASF(4) " : Outport  VectorParamsAs1DForOutWhenUnconnected=off
  wires:
  " "/1 -> lb-mol/h/2
  "  "/1 -> lb-mol/h/3
  XMEAS in kscmh/1 -> lb-mol/h/1
  Convert from lb/h to kg/h/1 -> Product/3
  XST/1 -> XMWS Molecular weight of Stream lb/lb-mol/1(XST)
  lb-mol/h/1 -> Product/2
  XMWS Molecular weight of Stream lb/lb-mol/1(XMWS) -> Product/1
  Product/1 -> "SMEASF(4) "/1  "SMEASF(4)"

== system COSTEP/Stream Measurements/Subsystem6/A and C feed stream/Pressure measurement in kPa ==
  "P in mm Hg " : Inport
  XMNSE : Inport  Port=2
  " kPa" : Constant  Value=101.325
  " mm Hg   " : Constant  Value=760
  Add : Sum
  Pressure conversion kPa : Product  Inputs=*/*
  SMEASP(4) : Outport  VectorParamsAs1DForOutWhenUnconnected=off
  wires:
  "P in mm Hg "/1 -> Pressure conversion kPa/1
  " kPa"/1 -> Pressure conversion kPa/3
  " mm Hg   "/1 -> Pressure conversion kPa/2
  Pressure conversion kPa/1 -> Add/1
  Add/1 -> SMEASP(4)/1  "SMEASP(4)"
  XMNSE/1 -> Add/2

== system COSTEP/Stream Measurements/Subsystem6/A and C feed stream/Temperature measurement in C ==
  T in celsius : Inport
  XMNSE : Inport  Port=2
  Add : Sum
  SMEAST(4) : Outport
  wires:
  T in celsius/1 -> Add/1
  Add/1 -> SMEAST(4)/1  "SMEAST"
  XMNSE/1 -> Add/2

== system COSTEP/Stream Measurements/Subsystem6/A feed stream/Composition measurement mol% ==
  XST : Inport
  XMNSE : Inport  Port=2
  Bus Creator : BusCreator  Inputs=2
  Subsystem : Subsystem
  SMEASX(1) : Outport
  wires:
  XST/1 -> Subsystem/1(XST)
  Subsystem/2(SMEASXB(1)) -> Bus Creator/2  "SMEASXB(1)"
  Subsystem/1(SMEASXA(1)) -> Bus Creator/1  "SMEASXA(1)"
  Bus Creator/1 -> SMEASX(1)/1  "SMEASX(1)"
  XMNSE/1 -> Subsystem/2(XMNSE)

== system COSTEP/Stream Measurements/Subsystem6/A feed stream/Flow measurement in kg//h ==
  XMEAS in kscmh : Inport
  XST : Inport  Port=2
  " " : Constant  Value=35.3145
  "  " : Constant  Value=0.359
  Convert from lb/h to kg/h : Constant  Value=0.454
  XMWS Molecular weight of Stream lb/lb-mol : Subsystem
  kg/h : Product  Inputs=3
  lb-mol/h : Product  Inputs=**/
  "SMEASF(1) " : Outport  VectorParamsAs1DForOutWhenUnconnected=off
  wires:
  " "/1 -> lb-mol/h/2
  "  "/1 -> lb-mol/h/3
  XMEAS in kscmh/1 -> lb-mol/h/1
  Convert from lb/h to kg/h/1 -> kg/h/3
  XST/1 -> XMWS Molecular weight of Stream lb/lb-mol/1(XST)
  lb-mol/h/1 -> kg/h/2
  XMWS Molecular weight of Stream lb/lb-mol/1(XMWS) -> kg/h/1
  kg/h/1 -> "SMEASF(1) "/1

== system COSTEP/Stream Measurements/Subsystem6/A feed stream/Pressure measurement in kPa ==
  "P in mm Hg " : Inport
  XMNSE : Inport  Port=2
  " kPa" : Constant  Value=101.325
  " mm Hg   " : Constant  Value=760
  Add : Sum
  Pressure conversion kPa : Product  Inputs=*/*
  SMEASP(1) : Outport  VectorParamsAs1DForOutWhenUnconnected=off
  wires:
  "P in mm Hg "/1 -> Pressure conversion kPa/1
  " kPa"/1 -> Pressure conversion kPa/3
  " mm Hg   "/1 -> Pressure conversion kPa/2
  Pressure conversion kPa/1 -> Add/1
  Add/1 -> SMEASP(1)/1  "SMEASP"
  XMNSE/1 -> Add/2

== system COSTEP/Stream Measurements/Subsystem6/A feed stream/Temperature measurement in C ==
  T in celsius : Inport
  XMNSE : Inport  Port=2
  Add : Sum
  SMEAST(1) : Outport
  wires:
  T in celsius/1 -> Add/1
  Add/1 -> SMEAST(1)/1  "SMEAST"
  XMNSE/1 -> Add/2

== system COSTEP/Stream Measurements/Subsystem6/CCIn/Flow measurement in kg//h ==
  XMNSE : Inport
  F in gpm : Inport  Port=2
  Add : Sum
  Product : Product
  Product1 : Product
  gpm to lb/h : Constant  Value=500.72
  kg/kmol : Constant  Value=18.02
  kmol : Constant  Value=0.45359237
  kmol/h : Product
  lb/h to lb-mol/h : Product  Inputs=*/
  lb/lb-mol : Constant  Value=18.02
  "SMEASF " : Outport  VectorParamsAs1DForOutWhenUnconnected=off
  wires:
  Add/1 -> "SMEASF "/1  "SMEASF"
  Product/1 -> Add/1
  XMNSE/1 -> Add/2
  Product1/1 -> lb/h to lb-mol/h/1
  lb/lb-mol/1 -> lb/h to lb-mol/h/2
  lb/h to lb-mol/h/1 -> kmol/h/2
  gpm to lb/h/1 -> Product1/2
  F in gpm/1 -> Product1/1
  kmol/1 -> kmol/h/1
  kmol/h/1 -> Product/1
  kg/kmol/1 -> Product/2

== system COSTEP/Stream Measurements/Subsystem6/CCIn/Pressure measurement in kPa ==
  XMNSE : Inport
  TC : Inport  Port=2
  A Antoine Coefficient A : Constant  Value=11.6834
  Add : Sum
  Add1 : Sum
  Add2 : Sum  Inputs=+-
  B Antoine Coefficient B : Constant  Value=3816.44
  C Antoine Coefficient C : Constant  Value=-46.13
  Divide : Product  Inputs=*/
  Divide1 : Product  Inputs=**
  Math Function : Math  SignedPower=on
  Temperature in Kelvin K : Sum
  To Convert bar to kPa : Constant  Value=100
  To Convert °C to K : Constant  Value=273.15
  SMEASP : Outport  VectorParamsAs1DForOutWhenUnconnected=off
  wires:
  Add/1 -> SMEASP/1  "SMEASP"
  XMNSE/1 -> Add/2
  To Convert °C to K/1 -> Temperature in Kelvin K/2
  TC/1 -> Temperature in Kelvin K/1
  C Antoine Coefficient C/1 -> Add1/1
  Divide/1 -> Add2/2
  B Antoine Coefficient B/1 -> Divide/1
  Add1/1 -> Divide/2
  Math Function/1 -> Divide1/1
  A Antoine Coefficient A/1 -> Add2/1
  Add2/1 -> Math Function/1
  To Convert bar to kPa/1 -> Divide1/2
  Temperature in Kelvin K/1 -> Add1/2
  Divide1/1 -> Add/1

== system COSTEP/Stream Measurements/Subsystem6/CCIn/Temperature measurement in C ==
  T in celsius : Inport
  XMNSE : Inport  Port=2
  Add : Sum
  SMEAST : Outport
  wires:
  T in celsius/1 -> Add/1
  Add/1 -> SMEAST/1  "SMEAST"
  XMNSE/1 -> Add/2

== system COSTEP/Stream Measurements/Subsystem6/CCOut/Pressure measurement in kPa ==
  XMNSE : Inport
  TC : Inport  Port=2
  A Antoine Coefficient A : Constant  Value=11.6834
  Add : Sum
  Add1 : Sum
  Add2 : Sum  Inputs=+-
  B Antoine Coefficient B : Constant  Value=3816.44
  C Antoine Coefficient C : Constant  Value=-46.13
  Divide : Product  Inputs=*/
  Divide1 : Product  Inputs=**
  Math Function : Math  SignedPower=on
  Temperature in Kelvin K : Sum
  To Convert bar to kPa : Constant  Value=100
  To Convert °C to K : Constant  Value=273.15
  SMEASP : Outport  VectorParamsAs1DForOutWhenUnconnected=off
  wires:
  Add/1 -> SMEASP/1  "SMEASP"
  XMNSE/1 -> Add/2
  To Convert °C to K/1 -> Temperature in Kelvin K/2
  TC/1 -> Temperature in Kelvin K/1
  C Antoine Coefficient C/1 -> Add1/1
  Divide/1 -> Add2/2
  B Antoine Coefficient B/1 -> Divide/1
  Add1/1 -> Divide/2
  Math Function/1 -> Divide1/1
  A Antoine Coefficient A/1 -> Add2/1
  Add2/1 -> Math Function/1
  To Convert bar to kPa/1 -> Divide1/2
  Temperature in Kelvin K/1 -> Add1/2
  Divide1/1 -> Add/1

== system COSTEP/Stream Measurements/Subsystem6/CCOut/Temperature measurement in C ==
  T in celsius : Inport
  XMNSE : Inport  Port=2
  Add : Sum
  SMEAST : Outport
  wires:
  T in celsius/1 -> Add/1
  Add/1 -> SMEAST/1  "SMEAST"
  XMNSE/1 -> Add/2

== system COSTEP/Stream Measurements/Subsystem6/Condenser product stream/Composition measurement mol% ==
  XST : Inport
  XMNSE : Inport  Port=2
  Bus Creator : BusCreator  Inputs=8
  Subsystem : Subsystem
  SMEASX : Outport
  wires:
  Subsystem/4(SMEASXD) -> Bus Creator/4  "SMEASXD"
  Subsystem/5(SMEASXE) -> Bus Creator/5  "SMEASXE"
  Subsystem/6(SMEASXF) -> Bus Creator/6  "SMEASXF"
  Subsystem/7(SMEASXG) -> Bus Creator/7  "SMEASXG"
  Subsystem/8(SMEASXH) -> Bus Creator/8  "SMEASXH"
  Subsystem/3(SMEASXC) -> Bus Creator/3  "SMEASXC"
  XST/1 -> Subsystem/1(XST)
  Subsystem/2(SMEASXB) -> Bus Creator/2  "SMEASXB"
  Subsystem/1(SMEASXA) -> Bus Creator/1  "SMEASXA"
  Bus Creator/1 -> SMEASX/1  "SMEASX"
  XMNSE/1 -> Subsystem/2(XMNSE)

== system COSTEP/Stream Measurements/Subsystem6/Condenser product stream/Flow measurement in kg//h ==
  XST : Inport
  XMNSE : Inport  Port=2
  F in lb-mol/h : Inport  Port=3
  Add : Sum
  Convert from lb/h to kg/h : Constant  Value=0.454
  Product : Product  Inputs=3
  XMWS Molecular weight of Stream lb/lb-mol : Subsystem
  "SMEASF " : Outport  VectorParamsAs1DForOutWhenUnconnected=off
  wires:
  Convert from lb/h to kg/h/1 -> Product/3
  Add/1 -> "SMEASF "/1  "SMEASF"
  Product/1 -> Add/1
  XST/1 -> XMWS Molecular weight of Stream lb/lb-mol/1(XST)
  XMWS Molecular weight of Stream lb/lb-mol/1(XMWS) -> Product/1
  XMNSE/1 -> Add/2
  F in lb-mol/h/1 -> Product/2

== system COSTEP/Stream Measurements/Subsystem6/Condenser product stream/Pressure measurement in kPa ==
  XMEAS in kPa gauge : Inport
  " kPa" : Constant  Value=101.325
  Add : Sum
  SMEASP : Outport  VectorParamsAs1DForOutWhenUnconnected=off
  wires:
  Add/1 -> SMEASP/1  "SMEASP"
  " kPa"/1 -> Add/2
  XMEAS in kPa gauge/1 -> Add/1

== system COSTEP/Stream Measurements/Subsystem6/Condenser product stream/Subsystem ==
  HST(8) : Inport
  XST : Inport  Port=2
  ITY : Inport  Port=3
  "  " : Product  Inputs=*/
  "HST(8a) " : Sum
  Product1 : Product
  "TST(8a) Temperature of Stream °C " : Subsystem
  gpm to lb/h : Constant  Value=500.72
  lb/h to lb-mol/h : Product  Inputs=*/
  lb/lb-mol : Constant  Value=18.02
  TST(8a) : Outport
  wires:
  lb/h to lb-mol/h/1 -> "  "/2
  Product1/1 -> lb/h to lb-mol/h/1
  ITY/1 -> "TST(8a) Temperature of Stream °C "/3(ITY)
  gpm to lb/h/1 -> Product1/2
  "  "/1 -> "HST(8a) "/2
  [FWS] -> Product1/1
  HST(8)/1 -> "HST(8a) "/1
  "HST(8a) "/1 -> "TST(8a) Temperature of Stream °C "/1(HST)  "HST(8a)"
  lb/lb-mol/1 -> lb/h to lb-mol/h/2
  XST/1 -> "TST(8a) Temperature of Stream °C "/2(XLR)
  [QUS] -> "  "/1
  "TST(8a) Temperature of Stream °C "/1(TST(8a)) -> TST(8a)/1

== system COSTEP/Stream Measurements/Subsystem6/Condenser product stream/Temperature measurement in C ==
  XMEAS in celsius : Inport
  SMEAST : Outport
  wires:
  XMEAS in celsius/1 -> SMEAST/1  "SMEAST"

== system COSTEP/Stream Measurements/Subsystem6/D feed stream/Composition measurement mol% ==
  XST : Inport
  XMNSE : Inport  Port=2
  Bus Creator : BusCreator  Inputs=2
  Subsystem : Subsystem
  SMEASX(2) : Outport
  wires:
  XST/1 -> Subsystem/1(XST)
  Bus Creator/1 -> SMEASX(2)/1  "SMEASX(2)"
  XMNSE/1 -> Subsystem/2(XMNSE)
  Subsystem/1(SMEASXB(2)) -> Bus Creator/1  "SMEASXB(2)"
  Subsystem/2(SMEASXD(2)) -> Bus Creator/2  "SMEASXD(2)"

== system COSTEP/Stream Measurements/Subsystem6/D feed stream/Flow measurement in kg//h ==
  XMEAS in kg/h : Inport
  "SMEASF(2) " : Outport  VectorParamsAs1DForOutWhenUnconnected=off
  wires:
  XMEAS in kg/h/1 -> "SMEASF(2) "/1

== system COSTEP/Stream Measurements/Subsystem6/D feed stream/Pressure measurement in kPa ==
  "P in mm Hg " : Inport
  XMNSE : Inport  Port=2
  " kPa" : Constant  Value=101.325
  " mm Hg   " : Constant  Value=760
  Add : Sum
  Pressure conversion kPa : Product  Inputs=*/*
  SMEASP(2) : Outport  VectorParamsAs1DForOutWhenUnconnected=off
  wires:
  "P in mm Hg "/1 -> Pressure conversion kPa/1
  " kPa"/1 -> Pressure conversion kPa/3
  " mm Hg   "/1 -> Pressure conversion kPa/2
  Pressure conversion kPa/1 -> Add/1
  Add/1 -> SMEASP(2)/1  "SMEASP"
  XMNSE/1 -> Add/2

== system COSTEP/Stream Measurements/Subsystem6/D feed stream/Temperature measurement in C ==
  T in celsius : Inport
  XMNSE : Inport  Port=2
  Add : Sum
  SMEAST(2) : Outport
  wires:
  T in celsius/1 -> Add/1
  Add/1 -> SMEAST(2)/1  "SMEAST"
  XMNSE/1 -> Add/2

== system COSTEP/Stream Measurements/Subsystem6/E feed stream/Composition measurement mol% ==
  XST : Inport
  XMNSE : Inport  Port=2
  Bus Creator : BusCreator  Inputs=2
  Subsystem : Subsystem
  SMEASX(3) : Outport
  wires:
  Subsystem/1(SMEASXE(3)) -> Bus Creator/1  "SMEASXE(3)"
  Subsystem/2(SMEASXF(3)) -> Bus Creator/2  "SMEASXF(3)"
  XST/1 -> Subsystem/1(XST)
  Bus Creator/1 -> SMEASX(3)/1  "SMEASX(3)"
  XMNSE/1 -> Subsystem/2(XMNSE)

== system COSTEP/Stream Measurements/Subsystem6/E feed stream/Flow measurement in kg//h ==
  XMEAS in kg/h : Inport
  "SMEASF(3) " : Outport  VectorParamsAs1DForOutWhenUnconnected=off
  wires:
  XMEAS in kg/h/1 -> "SMEASF(3) "/1

== system COSTEP/Stream Measurements/Subsystem6/E feed stream/Pressure measurement in kPa ==
  "P in mm Hg " : Inport
  XMNSE : Inport  Port=2
  " kPa" : Constant  Value=101.325
  " mm Hg   " : Constant  Value=760
  Add : Sum
  Pressure conversion kPa : Product  Inputs=*/*
  SMEASP(3) : Outport  VectorParamsAs1DForOutWhenUnconnected=off
  wires:
  "P in mm Hg "/1 -> Pressure conversion kPa/1
  " kPa"/1 -> Pressure conversion kPa/3
  " mm Hg   "/1 -> Pressure conversion kPa/2
  Pressure conversion kPa/1 -> Add/1
  Add/1 -> SMEASP(3)/1  "SMEASP"
  XMNSE/1 -> Add/2

== system COSTEP/Stream Measurements/Subsystem6/E feed stream/Temperature measurement in C ==
  T in celsius : Inport
  XMNSE : Inport  Port=2
  Add : Sum
  SMEAST(3) : Outport
  wires:
  T in celsius/1 -> Add/1
  Add/1 -> SMEAST(3)/1  "SMEAST"
  XMNSE/1 -> Add/2

== system COSTEP/Stream Measurements/Subsystem6/Product stream/Composition measurement mol% ==
  XST : Inport
  XMNSE2 : Inport  Port=2
  XMNSE3 : Inport  Port=3
  Bus Creator : BusCreator  Inputs=8
  Subsystem : Subsystem
  Subsystem1 : Subsystem
  SMEASX : Outport
  wires:
  Subsystem/3(SMEASXC) -> Bus Creator/3  "SMEASXC"
  XST/1 -> Subsystem1/1(XST), Subsystem/1(XST)
  Subsystem/2(SMEASXB) -> Bus Creator/2  "SMEASXB"
  Subsystem/1(SMEASXA) -> Bus Creator/1  "SMEASXA"
  Bus Creator/1 -> SMEASX/1  "SMEASX"
  XMNSE2/1 -> Subsystem/2(XMNSE)
  Subsystem1/1(SMEASXD) -> Bus Creator/4  "SMEASXD"
  Subsystem1/2(SMEASXE) -> Bus Creator/5  "SMEASXE"
  Subsystem1/3(SMEASXF) -> Bus Creator/6  "SMEASXF"
  Subsystem1/4(SMEASXG) -> Bus Creator/7  "SMEASXG"
  Subsystem1/5(SMEASXH) -> Bus Creator/8  "SMEASXH"
  XMNSE3/1 -> Subsystem1/2(XMNSE3)

== system COSTEP/Stream Measurements/Subsystem6/Product stream/Flow measurement in kg//h ==
  XMEAS in m^3/h : Inport
  XST : Inport  Port=2
  "       " : Constant  Value=35.3145
  Convert from lb/h to kg/h : Constant  Value=0.454
  XMWS Molecular weight of Stream lb/lb-mol : Subsystem
  kg/h : Product  Inputs=3
  lb-mol/h : Product  Inputs=***
  "SMEASF " : Outport  VectorParamsAs1DForOutWhenUnconnected=off
  wires:
  lb-mol/h/1 -> kg/h/2
  [DLS] -> lb-mol/h/2
  "       "/1 -> lb-mol/h/3
  XMEAS in m^3/h/1 -> lb-mol/h/1
  XMWS Molecular weight of Stream lb/lb-mol/1(XMWS) -> kg/h/1
  Convert from lb/h to kg/h/1 -> kg/h/3
  kg/h/1 -> "SMEASF "/1
  XST/1 -> XMWS Molecular weight of Stream lb/lb-mol/1(XST)

== system COSTEP/Stream Measurements/Subsystem6/Product stream/Pressure measurement in kPa ==
  "P in mm Hg " : Inport
  XMNSE : Inport  Port=2
  " kPa" : Constant  Value=101.325
  " mm Hg   " : Constant  Value=760
  Add : Sum
  Pressure conversion kPa : Product  Inputs=*/*
  SMEASP : Outport  VectorParamsAs1DForOutWhenUnconnected=off
  wires:
  "P in mm Hg "/1 -> Pressure conversion kPa/1
  " kPa"/1 -> Pressure conversion kPa/3
  " mm Hg   "/1 -> Pressure conversion kPa/2
  Pressure conversion kPa/1 -> Add/1
  Add/1 -> SMEASP/1  "SMEASP"
  XMNSE/1 -> Add/2
